simulink model "cascade_realizationsubsystem"  (R2020a)
settings: Solver=FixedStepAuto  StartTime=0.0  StopTime=10.0  FixedStep=0.2  RelTol=1e-3
settings Model: Creator=Jake  LastModifiedBy=Jake
settings DataIOCC: SaveOutput=off  SaveTime=off

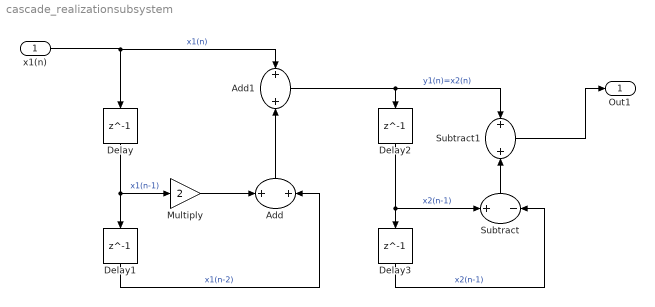
== system cascade_realizationsubsystem ==
  x1(n) : Inport  OutDataTypeStr=double  PortDimensions=1  SampleTime=[0.20000000000000001,0]
  Add : Sum
  Add1 : Sum
  Delay{,1..3} (4 alike) : Delay  DelayLength=1
  Multiply : Gain  Gain=2
  Subtract : Sum  Inputs=+-
  Subtract1 : Sum
  Out1 : Outport  OutDataTypeStr=double  PortDimensions=1  SampleTime=[0.20000000000000001,0]
  wires:
  Subtract/1 -> Subtract1/2
  Delay2/1 -> Subtract/1, Delay3/1  "x2(n-1)"
  Multiply/1 -> Add/1
  Delay1/1 -> Add/2  "x1(n-2)"
  x1(n)/1 -> Delay/1, Add1/1  "x1(n)"
  Delay/1 -> Delay1/1, Multiply/1  "x1(n-1)"
  Add1/1 -> Subtract1/1, Delay2/1  "y1(n)=x2(n)"
  Add/1 -> Add1/2
  Delay3/1 -> Subtract/2  "x2(n-1)"
  Subtract1/1 -> Out1/1
